simulink model "MPC_SinCasadi_V1_2016b"  (R2018b)
settings: Solver=ode4  StartTime=0.0  StopTime=inf  FixedStep=Ts  RelTol=1e-3
PreLoadFcn:
  | %% Parametros Simulacion %%
  | Ts = 50e-5; % tiempo simulacion
  | Tc = 2e-3;  % tiempo control
  | % Voltaje Nominal
  | vnom = 380;
  | % # de nodos
  | n = 4;
  | nic = 100;
  | pasoc = 0.1;
  | pv = 0.01;
  | px = 0.1;
  | 
  | % parametros de resistencia
  | r = [0.0226 0.0257 0.0769 0.0164 0.0513 0.0164 0.0411];
  | %Potencia Disponible
  | P = 100000;
  | %Bases de conversion
  | Vbase = 380;
  | Pbase = 1000;
  | %Filtros Droop
  | T = 0.5;
  | T1 = T;
  | T2 = T;
  | T3 = T;
  | T4 = T;
  | % Parametros del Droop
  | z1 = 0.0005527;
  | z2 = 0.0020;
  | z3 = 0.0017;
  | z4 = 0.0008107;
  | % Inicializacion Potencia y estados
  | Pi = 0.25;
  | xi = [Pi;Pi;Pi;Pi]*P;
  | % Filtro Potencia Disponible
  | Tf = 0.1;
  | % Filtro Control
  | Tfilter = 0.1;
InitFcn:
  | %% Parametros Simulacion %%
  | Ts = 50e-5; % tiempo simulacion
  | Tc = 2e-3;  % tiempo control
  | % Voltaje Nominal
  | vnom = 380;
  | % # de nodos
  | n = 4;
  | nic = 100;
  | pasoc = 0.1;
  | pv = 0.01;
  | px = 0.1;
  | 
  | % parametros de resistencia
  | r = [0.0226 0.0257 0.0769 0.0164 0.0513 0.0164 0.0411];
  | %Potencia Disponible
  | P = 100000;
  | %Bases de conversion
  | Vbase = 380;
  | Pbase = 1000;
  | %Filtros Droop
  | T = 0.5;
  | T1 = T;
  | T2 = T;
  | T3 = T;
  | T4 = T;
  | % Parametros del Droop
  | z1 = 0.0005527;
  | z2 = 0.0020;
  | z3 = 0.0017;
  | z4 = 0.0008107;
  | % Inicializacion Potencia y estados
  | Pi = 0.25;
  | xi = [Pi;Pi;Pi;Pi]*P;
  | % Filtro Potencia Disponible
  | Tf = 0.1;
  | % Filtro Control
  | Tfilter = 0.1;
undefined symbols (not defined in the file or in its folder): another_event_name, my_event_name
libraries: powerlib x38, rtlab x4, rtio_opalrt_common x3, simulink x1
settings Model: Creator=santi  LastModifiedBy=aperez
settings DataIOCC: ReturnWorkspaceOutputs=on
settings OptimizationCC: DefaultParameterBehavior=Inlined
settings DebuggingCC: UnconnectedInputMsg=none  UnconnectedOutputMsg=none  UnconnectedLineMsg=none  SFMachineParentedDataDiag=error
settings HardwareCC: TargetBitPerPointer=64  TargetBitPerSizeT=64  TargetBitPerPtrDiffT=64  TargetLongLongMode=on  TargetIntDivRoundTo=Zero  TargetEndianess=LittleEndian  TargetWordSize=64  TargetHWDeviceType=MATLAB Host  ProdEqTarget=off
settings ModelReferenceCC: EnableRefExpFcnMdlSchedulingChecks=off
settings RTWCC: SystemTargetFile=rtwsfcn.tlc  TemplateMakefile=rtwsfcn_default_tmf  Description=S-Function Target
settings CodeAppCC: StateflowObjectComments=on
settings STFCustomTargetCC: TargetLangStandard=C99 (ISO)  ModelReferenceCompliant=off  CompOptLevelCompliant=on  MATLABClassNameForMDSCustomization=Simulink.SoftwareTarget.TargetSpecificTriggerConfigurationBase  GRTInterface=on  SystemTargetFile=rtwsfcn.tlc

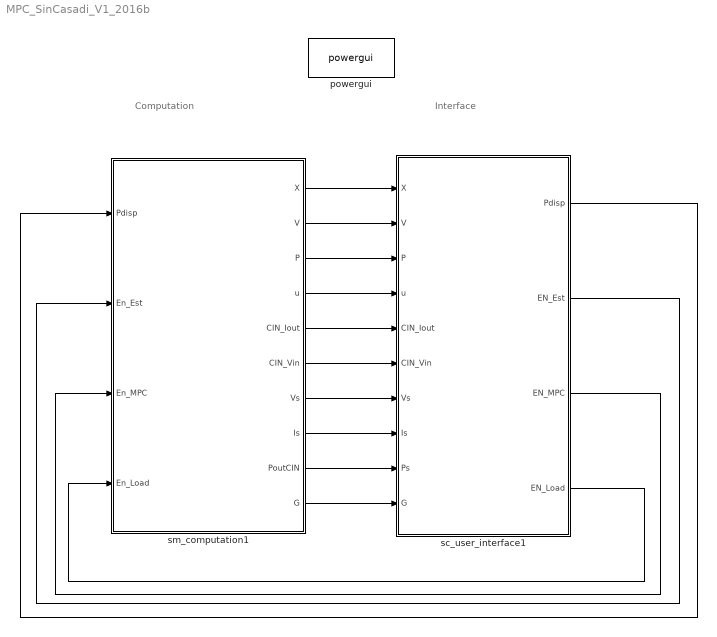
== system MPC_SinCasadi_V1_2016b ==
  note: Computation
  note: Interface
  powergui : powerlib/powergui  Priority=1  SimulationMode=Discrete  SampleTime=Ts  frequency=60  Iterations=50  frequencyindice=0  Pbase=100e6  ErrMax=1e-4  UnitsV=kV  UnitsW=MW  buscounter=0  FunctionMessages=off  echomessages=off  EnableUseOfTLC=off  CurrentSourceSwitches=off  DisableSnubberDevices=off  DisableRonSwitches=off  DisableVfSwitches=off  DisplayEquations=off  SolverType=Tustin/Backward Euler (TBE)  Interpol=off  ExternalGateDelay=off  methode=off  Ts=10  x0status=blocks  SPID=off  SwTol=0  HookPort=off  RestoreLinks=warning  ResistiveCurrentMeasurement=off  Frange=[0:2:500]  Ylog=off  Xlog=on  ShowGrid=off  save=off  variable=ZData  structure=0  ZoomFFT=off  StartTime=0.0  cycles=1  DisplayStyle=1  fundamental=60  FreqAxis=off  MaxFrequency=1000  frequencyindicesteady=1  RmsSteady=1  display=off
  sc_user_interface1 : Subsystem
  sm_computation1 : Subsystem
  wires:
  sc_user_interface1/1("Pdisp ") -> sm_computation1/1(Pdisp)
  sm_computation1/2(V) -> sc_user_interface1/2(V)
  sm_computation1/3(P) -> sc_user_interface1/3(P)
  sm_computation1/1(X) -> sc_user_interface1/1(X)
  sm_computation1/4(u) -> sc_user_interface1/4(u)
  sm_computation1/5(CIN_Iout) -> sc_user_interface1/5(CIN_Iout)
  sm_computation1/6(CIN_Vin) -> sc_user_interface1/6(CIN_Vin)
  sm_computation1/7(Vs) -> sc_user_interface1/7(Vs)
  sm_computation1/8(Is) -> sc_user_interface1/8(Is)
  sm_computation1/9(PoutCIN) -> sc_user_interface1/9(Ps)
  sm_computation1/10(G) -> sc_user_interface1/10(G)
  sc_user_interface1/2("EN_Est ") -> sm_computation1/2(En_Est)
  sc_user_interface1/3(EN_MPC) -> sm_computation1/3(En_MPC)
  sc_user_interface1/4("EN_Load ") -> sm_computation1/4(En_Load)

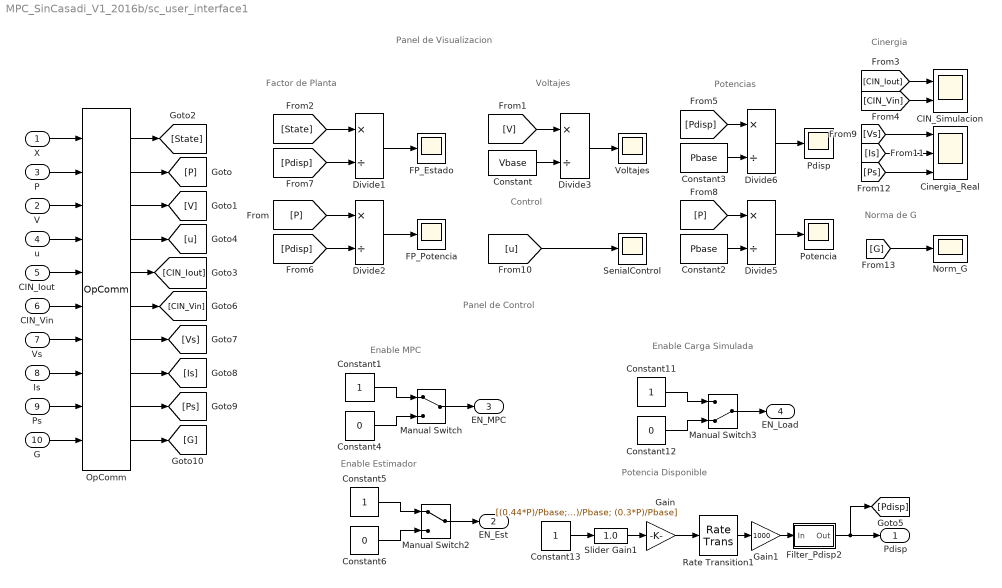
== system MPC_SinCasadi_V1_2016b/sc_user_interface1 ==
  note: Factor de Planta
  note: Potencias
  note: Voltajes
  note: Potencia Disponible
  note: Control
  note: Panel de Visualizacion
  note: Enable MPC
  note: Enable Estimador
  note: Enable Carga Simulada
  note: Panel de Control
  note: Cinergia
  note: Norma de G
  X : Inport
  V : Inport  Port=2
  P : Inport  Port=3
  u : Inport  Port=4
  CIN_Iout : Inport  Port=5
  CIN_Vin : Inport  Port=6
  Vs : Inport  Port=7
  Is : Inport  Port=8
  Ps : Inport  Port=9
  G : Inport  Port=10
  CIN_Simulacion : Scope  NumInputPorts=2
  Cinergia_Real : Scope  NumInputPorts=3
  Constant : Constant  Value=Vbase
  Constant{1,5,11,13} (4 alike) : Constant
  Constant12 : Constant  Value=0
  Constant2 : Constant  Value=Pbase
  Constant3 : Constant  Value=Pbase
  Constant4 : Constant  Value=0
  Constant6 : Constant  Value=0
  Divide{1..3,5..6} (5 alike) : Product  Inputs=*/
  FP_Estado : Scope
  FP_Potencia : Scope
  Filter_Pdisp2 : Subsystem
  Gain : Gain  Gain=[(0.44*P)/Pbase; (0.12*P)/Pbase; (0.14*P)/Pbase; (0.3*P)/Pbase]
  Gain1 : Gain  Gain=1000
  Manual Switch : ManualSwitch
  Manual Switch2 : ManualSwitch
  Manual Switch3 : ManualSwitch  CurrentSetting=0
  Norm_G : Scope
  OpComm : rtlab/OpComm  nbport=10  groupe_acq=1  subsys_rate=0  st=0  Synchronization=on  Interpolation=on  Threshold=1.0  Missed_Data=off  Sim_Time=off  Samples=off  dynSigOut=off  from_console=0  warning_done=off  writeOpCommFile=off  Offset=off
  Pdisp : Scope
  Potencia : Scope
  Rate Transition1 : RateTransition  InitialCondition=[45;12;20;30]  OutPortSampleTime=Tc
  SenialControl : Scope
  Slider Gain1 : simulink/Math Operations/Slider Gain  gain=1.0  low=0.4  high=1
  Voltajes : Scope
  "Pdisp " : Outport
  "EN_Est " : Outport  Port=2
  EN_MPC : Outport  Port=3
  "EN_Load " : Outport  Port=4
  wires:
  [P] -> Divide2/1
  Divide2/1 -> FP_Potencia/1
  Divide1/1 -> FP_Estado/1
  Divide3/1 -> Voltajes/1
  [V] -> Divide3/1
  Constant/1 -> Divide3/2
  [State] -> Divide1/1
  [Pdisp] -> Divide2/2
  [Pdisp] -> Divide1/2
  [P] -> Divide5/1
  Divide5/1 -> Potencia/1
  [u] -> SenialControl/1
  Constant2/1 -> Divide5/2
  Divide6/1 -> Pdisp/1
  Constant3/1 -> Divide6/2
  [Pdisp] -> Divide6/1
  X/1 -> OpComm/1
  P/1 -> OpComm/2
  V/1 -> OpComm/3
  OpComm/3 -> [V]
  OpComm/2 -> [P]
  OpComm/1 -> [State]
  OpComm/4 -> [u]
  u/1 -> OpComm/4
  Gain1/1 -> Filter_Pdisp2/1(In)
  Gain/1 -> Rate Transition1/1
  Filter_Pdisp2/1(Out) -> "Pdisp "/1, [Pdisp]
  Rate Transition1/1 -> Gain1/1
  CIN_Iout/1 -> OpComm/5
  CIN_Vin/1 -> OpComm/6
  Vs/1 -> OpComm/7
  Is/1 -> OpComm/8
  Ps/1 -> OpComm/9
  G/1 -> OpComm/10
  Constant1/1 -> Manual Switch/1
  Constant4/1 -> Manual Switch/2
  Manual Switch/1 -> EN_MPC/1
  Manual Switch2/1 -> "EN_Est "/1
  Constant6/1 -> Manual Switch2/2
  Constant5/1 -> Manual Switch2/1
  Constant11/1 -> Manual Switch3/1
  Constant12/1 -> Manual Switch3/2
  Manual Switch3/1 -> "EN_Load "/1
  Slider Gain1/1 -> Gain/1
  Constant13/1 -> Slider Gain1/1
  OpComm/5 -> [CIN_Iout]
  OpComm/6 -> [CIN_Vin]
  OpComm/7 -> [Vs]
  OpComm/8 -> [Is]
  OpComm/9 -> [Ps]
  OpComm/10 -> [G]
  [G] -> Norm_G/1
  [Vs] -> Cinergia_Real/1
  [Is] -> Cinergia_Real/2
  [Ps] -> Cinergia_Real/3
  [CIN_Vin] -> CIN_Simulacion/2
  [CIN_Iout] -> CIN_Simulacion/1

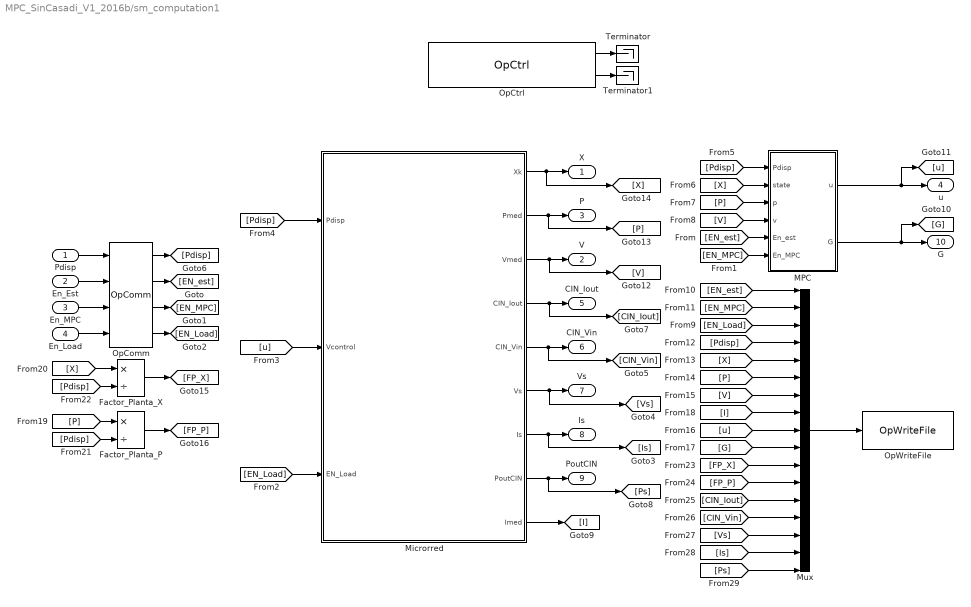
== system MPC_SinCasadi_V1_2016b/sm_computation1 ==
  Pdisp : Inport
  En_Est : Inport  Port=2
  En_MPC : Inport  Port=3
  En_Load : Inport  Port=4
  Factor_Planta_P : Product  Inputs=*/
  Factor_Planta_X : Product  Inputs=*/
  MPC : Subsystem
  Microrred : Subsystem
      settings: MinAlgLoopOccurrences=on
  Mux : Mux  Inputs=17
  OpComm : rtlab/OpComm  nbport=4  groupe_acq=1  subsys_rate=0  st=0  Synchronization=on  Interpolation=on  Threshold=1.0  Missed_Data=off  Sim_Time=off  Samples=off  dynSigOut=off  from_console=1  warning_done=off  writeOpCommFile=off  Offset=off
  OpCtrl : rtio_opalrt_common/OpCtrl  CtrlName='OpCtrl'  boardid=0  BitstreamFilename=VC707_2-EX-0001-3_2_3_354-eHSx128_C3C1FBCEC3C3FBFB-FF-01.bin  numconfig=-1  mode=Master  externalClock=off  decimRtsi=0  calibIO=off  SampleTime=Ts  loadinport=-1  BoardType=VC707  SecondaryPresent=off  sync_type=Audio
  OpWriteFile : rtlab/DataLogging/OpWriteFile  Static_File=on  varname=opvar  Filename=myfile.mat  rtpath='./'  nrtpath='.\'  Acq_Group=26  file_size=[]  write_offline=off  Sim_Mode=off  Nb_Samples=1000  Buffer_size=1000000
  Terminator : Terminator
  Terminator1 : Terminator
  X : Outport
  V : Outport  Port=2
  P : Outport  Port=3
  u : Outport  Port=4
  CIN_Iout : Outport  Port=5
  CIN_Vin : Outport  Port=6
  Vs : Outport  Port=7
  Is : Outport  Port=8
  PoutCIN : Outport  Port=9
  G : Outport  Port=10
  wires:
  Microrred/1(Xk) -> X/1, [X]
  Microrred/2(Pmed) -> [P], P/1
  Microrred/3(Vmed) -> V/1, [V]
  Pdisp/1 -> OpComm/1
  OpComm/1 -> [Pdisp]
  OpCtrl/1 -> Terminator/1
  OpCtrl/2 -> Terminator1/1
  MPC/1(u) -> [u], u/1
  Microrred/4(CIN_Iout) -> [CIN_Iout], CIN_Iout/1
  Microrred/6(Vs) -> Vs/1, [Vs]
  Microrred/8(PoutCIN) -> PoutCIN/1, [Ps]
  MPC/2(G) -> [G], G/1
  Microrred/7(Is) -> Is/1, [Is]
  Microrred/5(CIN_Vin) -> CIN_Vin/1, [CIN_Vin]
  En_Est/1 -> OpComm/2
  En_MPC/1 -> OpComm/3
  OpComm/2 -> [EN_est]
  OpComm/3 -> [EN_MPC]
  [EN_est] -> MPC/5(En_est)
  [EN_MPC] -> MPC/6(En_MPC)
  En_Load/1 -> OpComm/4
  OpComm/4 -> [EN_Load]
  [EN_Load] -> Microrred/3(EN_Load)
  Microrred/9(Imed) -> [I]
  [u] -> Microrred/2(Vcontrol)
  [Pdisp] -> Microrred/1(Pdisp)
  [Pdisp] -> MPC/1(Pdisp)
  [X] -> MPC/2(state)
  [P] -> MPC/3(p)
  [V] -> MPC/4(v)
  Mux/1 -> OpWriteFile/1
  [EN_est] -> Mux/1
  [EN_MPC] -> Mux/2
  [EN_Load] -> Mux/3
  [Pdisp] -> Mux/4
  [X] -> Mux/5
  [P] -> Mux/6
  [V] -> Mux/7
  [I] -> Mux/8
  [u] -> Mux/9
  [G] -> Mux/10
  [X] -> Factor_Planta_X/1
  [Pdisp] -> Factor_Planta_X/2
  [Pdisp] -> Factor_Planta_P/2
  [P] -> Factor_Planta_P/1
  Factor_Planta_X/1 -> [FP_X]
  Factor_Planta_P/1 -> [FP_P]
  [FP_X] -> Mux/11
  [FP_P] -> Mux/12
  [Ps] -> Mux/17
  [CIN_Iout] -> Mux/13
  [CIN_Vin] -> Mux/14
  [Vs] -> Mux/15
  [Is] -> Mux/16

== system MPC_SinCasadi_V1_2016b/sc_user_interface1/Filter_Pdisp2 ==
  In : Inport
  Demux : Demux
  Discrete Transfer Fcn{,1..3} (4 alike) : DiscreteTransferFcn  Denominator=[(Tf/Ts) -(Tf/Ts)+1]  InitialStates=0.25*P
  Mux7 : Mux
  Out : Outport
  wires:
  Demux/4 -> Discrete Transfer Fcn3/1
  Demux/3 -> Discrete Transfer Fcn2/1
  Discrete Transfer Fcn3/1 -> Mux7/4
  Demux/1 -> Discrete Transfer Fcn/1
  Discrete Transfer Fcn1/1 -> Mux7/2
  Demux/2 -> Discrete Transfer Fcn1/1
  Discrete Transfer Fcn/1 -> Mux7/1
  Discrete Transfer Fcn2/1 -> Mux7/3
  Mux7/1 -> Out/1
  In/1 -> Demux/1

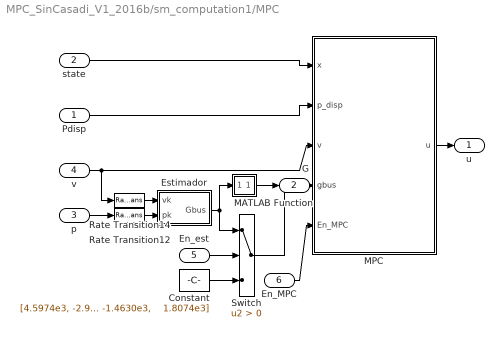
== system MPC_SinCasadi_V1_2016b/sm_computation1/MPC ==
  Pdisp : Inport
  state : Inport  Port=2
  p : Inport  Port=3
  v : Inport  Port=4
  En_est : Inport  Port=5
  En_MPC : Inport  Port=6
  Constant : Constant  Value="[4.5974e3, -2.9852e3, -1.2900e3, -0.3120e3; -2.9852e3, 2.9936e3, 0, 0; -1.2900e3,0,2.7560e3, -1.4630e3;   -0.3120e3,   0 ,  -1.4630e3,    1.8074e3]"
  Estimador : Subsystem
  MATLAB Function : MATLAB Function  TreatAsAtomicUnit=on
  MPC : Subsystem  TreatAsAtomicUnit=on  SystemSampleTime=Tc
      settings: MinAlgLoopOccurrences=on
  Rate Transition12 : RateTransition  InitialCondition=Pi*P  OutPortSampleTime=Tc
  Rate Transition14 : RateTransition  InitialCondition=[Vbase;Vbase;Vbase;Vbase]  OutPortSampleTime=Tc
  Switch : Switch  Criteria=u2 > Threshold
  u : Outport
  G : Outport  Port=2
  wires:
  Pdisp/1 -> MPC/2(p_disp)
  state/1 -> MPC/1(x)
  v/1 -> MPC/3(v), Rate Transition14/1
  p/1 -> Rate Transition12/1
  Rate Transition14/1 -> Estimador/1(vk)
  Rate Transition12/1 -> Estimador/2(pk)
  MPC/1(u) -> u/1
  En_est/1 -> Switch/2
  Switch/1 -> MPC/4(gbus)
  Estimador/1(Gbus) -> Switch/1, MATLAB Function/1(G)
  Constant/1 -> Switch/3
  MATLAB Function/1(normG) -> G/1
  En_MPC/1 -> MPC/5(En_MPC)

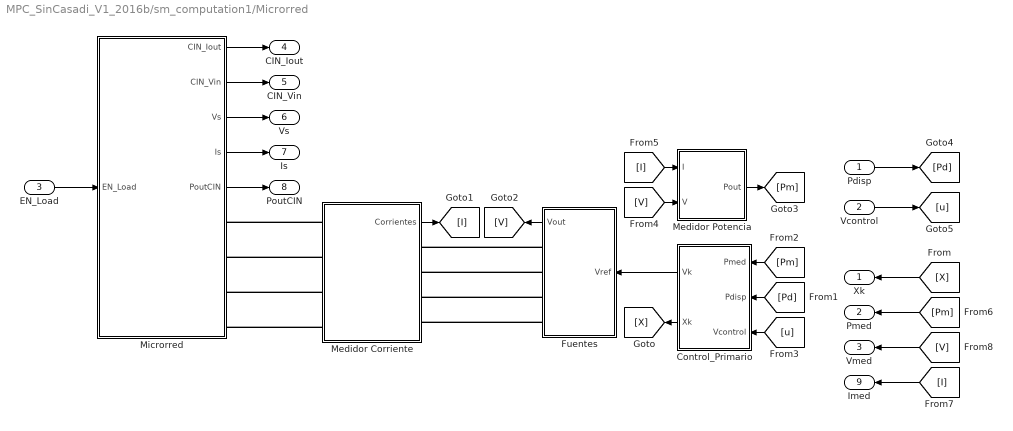
== system MPC_SinCasadi_V1_2016b/sm_computation1/Microrred ==
  Pdisp : Inport
  Vcontrol : Inport  Port=2
  EN_Load : Inport  Port=3
  Control_Primario : Subsystem
  Fuentes : Subsystem
  Medidor Corriente : Subsystem
  Medidor Potencia : Subsystem
  Microrred : Subsystem
  Xk : Outport
  Pmed : Outport  Port=2
  Vmed : Outport  Port=3
  CIN_Iout : Outport  Port=4
  CIN_Vin : Outport  Port=5
  Vs : Outport  Port=6
  Is : Outport  Port=7
  PoutCIN : Outport  Port=8
  Imed : Outport  Port=9
  wires:
  Control_Primario/1(Vk) -> Fuentes/1(Vref)
  Control_Primario/2(Xk) -> [X]
  Medidor Corriente/1(Corrientes) -> [I]
  Fuentes/1(Vout) -> [V]
  [Pd] -> Control_Primario/2(Pdisp)
  [Pm] -> Control_Primario/1(Pmed)
  [u] -> Control_Primario/3(Vcontrol)
  [V] -> Medidor Potencia/2(V)
  [I] -> Medidor Potencia/1(I)
  Medidor Potencia/1(Pout) -> [Pm]
  [X] -> Xk/1
  [Pm] -> Pmed/1
  [V] -> Vmed/1
  Pdisp/1 -> [Pd]
  Vcontrol/1 -> [u]
  Microrred/1(CIN_Iout) -> CIN_Iout/1
  Microrred/2(CIN_Vin) -> CIN_Vin/1
  Microrred/3(Vs) -> Vs/1
  Microrred/4(Is) -> Is/1
  Microrred/5(PoutCIN) -> PoutCIN/1
  EN_Load/1 -> Microrred/1(EN_Load)
  [I] -> Imed/1
  connections:
  Fuentes/RConn3 -- Medidor Corriente/RConn3
  Medidor Corriente/LConn3 -- Microrred/RConn3
  Fuentes/RConn4 -- Medidor Corriente/RConn4
  Medidor Corriente/LConn2 -- Microrred/RConn2
  Fuentes/RConn1 -- Medidor Corriente/RConn1
  Medidor Corriente/LConn1 -- Microrred/RConn1
  Fuentes/RConn2 -- Medidor Corriente/RConn2
  Medidor Corriente/LConn4 -- Microrred/RConn4

== system MPC_SinCasadi_V1_2016b/sm_computation1/MPC/Estimador ==
  vk : Inport
  pk : Inport  Port=2
  MATLAB System : MATLABSystem  System=Estimador_pu  Vbase=Vbase  Pbase=Pbase  SimulateUsing=Code generation
      mask Type: Estimador_pu
      mask Display:
      | disp('Estimador_pu');
      | port_label('input',1,'vk');
      | port_label('input',2,'pk');
      | port_label('output',1,'Gbus');
  Gbus : Outport
  wires:
  pk/1 -> MATLAB System/2
  vk/1 -> MATLAB System/1
  MATLAB System/1 -> Gbus/1

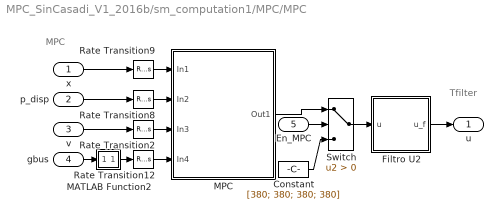
== system MPC_SinCasadi_V1_2016b/sm_computation1/MPC/MPC ==
  note: MPC
  note: Tfilter
  x : Inport
  p_disp : Inport  Port=2
  v : Inport  Port=3
  gbus : Inport  Port=4
  En_MPC : Inport  Port=5
  Constant : Constant  Value=[380; 380; 380; 380]
  Filtro U2 : Subsystem
  MATLAB Function2 : MATLAB Function  TreatAsAtomicUnit=on
  MPC : Subsystem  SystemSampleTime=2e-3
  Rate Transition12 : RateTransition  InitialCondition="[4.5974e3, -2.9852e3, -1.2900e3, -0.3120e3, -2.9852e3, 2.9936e3, 0, 0, -1.2900e3,0,2.7560e3, -1.4630e3,   -0.3120e3,   0 ,  -1.4630e3,    1.8074e3]"  OutPortSampleTime=Tc
  Rate Transition2 : RateTransition  InitialCondition=[Vbase;Vbase;Vbase;Vbase]  OutPortSampleTime=Tc
  Rate Transition8 : RateTransition  InitialCondition=Pi*P  OutPortSampleTime=Tc
  Rate Transition9 : RateTransition  InitialCondition=Pi*P  OutPortSampleTime=Tc
  Switch : Switch  Criteria=u2 > Threshold
  u : Outport
  wires:
  p_disp/1 -> Rate Transition8/1
  x/1 -> Rate Transition9/1
  v/1 -> Rate Transition2/1
  gbus/1 -> MATLAB Function2/1(gbus)
  Filtro U2/1(u_f) -> u/1
  Rate Transition9/1 -> MPC/1(In1)
  Rate Transition8/1 -> MPC/2(In2)
  Rate Transition2/1 -> MPC/3(In3)
  Rate Transition12/1 -> MPC/4(In4)
  MATLAB Function2/1(G) -> Rate Transition12/1
  MPC/1(Out1) -> Switch/1
  Switch/1 -> Filtro U2/1(u)
  Constant/1 -> Switch/3
  En_MPC/1 -> Switch/2

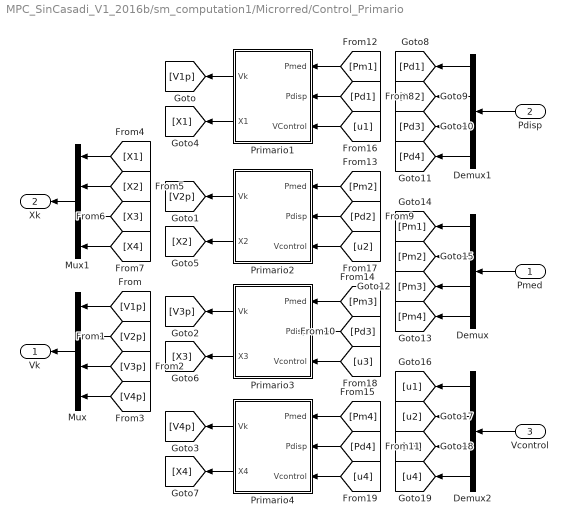
== system MPC_SinCasadi_V1_2016b/sm_computation1/Microrred/Control_Primario ==
  Pmed : Inport
  Pdisp : Inport  Port=2
  Vcontrol : Inport  Port=3
  Demux : Demux
  Demux1 : Demux
  Demux2 : Demux
  Mux : Mux
  Mux1 : Mux
  Primario1 : Subsystem
  Primario2 : Subsystem
  Primario3 : Subsystem
  Primario4 : Subsystem
  Vk : Outport
  Xk : Outport  Port=2
  wires:
  Vcontrol/1 -> Demux2/1
  Mux1/1 -> Xk/1
  Pmed/1 -> Demux/1
  Mux/1 -> Vk/1
  Pdisp/1 -> Demux1/1
  Primario1/1(Vk) -> [V1p]
  [V1p] -> Mux/1
  [V2p] -> Mux/2
  [V3p] -> Mux/3
  [V4p] -> Mux/4
  Primario2/1(Vk) -> [V2p]
  Primario3/1(Vk) -> [V3p]
  Primario4/1(Vk) -> [V4p]
  [X1] -> Mux1/1
  [X2] -> Mux1/2
  [X3] -> Mux1/3
  [X4] -> Mux1/4
  Primario2/2(X2) -> [X2]
  Primario3/2(X3) -> [X3]
  Primario4/2(X4) -> [X4]
  Primario1/2(X1) -> [X1]
  Demux1/1 -> [Pd1]
  Demux1/2 -> [Pd2]
  Demux1/3 -> [Pd3]
  Demux1/4 -> [Pd4]
  [Pd1] -> Primario1/2(Pdisp)
  [Pd2] -> Primario2/2(Pdisp)
  [Pd3] -> Primario3/2(Pdisp)
  [Pd4] -> Primario4/2(Pdisp)
  Demux/1 -> [Pm1]
  Demux/2 -> [Pm2]
  Demux/3 -> [Pm3]
  Demux/4 -> [Pm4]
  [Pm1] -> Primario1/1(Pmed)
  [Pm2] -> Primario2/1(Pmed)
  [Pm3] -> Primario3/1(Pmed)
  [Pm4] -> Primario4/1(Pmed)
  Demux2/1 -> [u1]
  Demux2/2 -> [u2]
  Demux2/3 -> [u3]
  Demux2/4 -> [u4]
  [u4] -> Primario4/3(Vcontrol)
  [u3] -> Primario3/3(Vcontrol)
  [u2] -> Primario2/3(Vcontrol)
  [u1] -> Primario1/3(VControl)

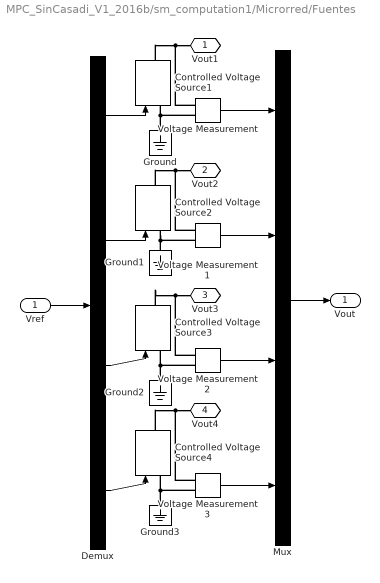
== system MPC_SinCasadi_V1_2016b/sm_computation1/Microrred/Fuentes ==
  Vref : Inport
  Controlled Voltage Source{1..4} (4 alike) : powerlib/Electrical Sources/Controlled Voltage Source  Initialize=on  Source_Type=DC  Amplitude=vnom  Phase=0  Frequency=0  Measurements=None
  Demux : Demux
  Ground{,1..3} (4 alike) : powerlib/Elements/Ground  LConnTagsString=a
  Mux : Mux
  Voltage Measurement{,1..3} (4 alike) : powerlib/Measurements/Voltage Measurement  PhasorSimulation=off  OutputType=Complex  PSBequivalent=0
  Vout1 : PMIOPort  Side=Right
  Vout2 : PMIOPort  Port=2  Side=Right
  Vout3 : PMIOPort  Port=3  Side=Right
  Vout4 : PMIOPort  Port=4  Side=Right
  Vout : Outport
  wires:
  Mux/1 -> Vout/1
  Voltage Measurement2/1 -> Mux/3
  Voltage Measurement1/1 -> Mux/2
  Voltage Measurement3/1 -> Mux/4
  Voltage Measurement/1 -> Mux/1
  Vref/1 -> Demux/1
  Demux/4 -> Controlled Voltage Source4/1
  Demux/3 -> Controlled Voltage Source3/1
  Demux/2 -> Controlled Voltage Source2/1
  Demux/1 -> Controlled Voltage Source1/1
  connections:
  Vout4/RConn1 -- Voltage Measurement3/LConn1 -- Controlled Voltage Source4/RConn1
  Voltage Measurement3/LConn2 -- Ground3/LConn1 -- Controlled Voltage Source4/LConn1
  Voltage Measurement2/LConn2 -- Ground2/LConn1 -- Controlled Voltage Source3/LConn1
  Vout3/RConn1 -- Voltage Measurement2/LConn1 -- Controlled Voltage Source3/RConn1
  Vout2/RConn1 -- Voltage Measurement1/LConn1 -- Controlled Voltage Source2/RConn1
  Voltage Measurement1/LConn2 -- Controlled Voltage Source2/LConn1 -- Ground1/LConn1
  Voltage Measurement/LConn2 -- Controlled Voltage Source1/LConn1 -- Ground/LConn1
  Vout1/RConn1 -- Voltage Measurement/LConn1 -- Controlled Voltage Source1/RConn1

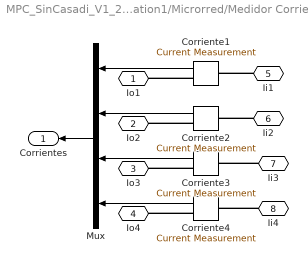
== system MPC_SinCasadi_V1_2016b/sm_computation1/Microrred/Medidor Corriente ==
  Corriente{1..4} (4 alike) : powerlib/Measurements/Current Measurement  PhasorSimulation=off  OutputType=Complex  PSBequivalent=0
  Mux : Mux
  Io1 : PMIOPort  Side=Left
  Io2 : PMIOPort  Port=2  Side=Left
  Io3 : PMIOPort  Port=3  Side=Left
  Io4 : PMIOPort  Port=4  Side=Left
  Ii1 : PMIOPort  Port=5  Side=Right
  Ii2 : PMIOPort  Port=6  Side=Right
  Ii3 : PMIOPort  Port=7  Side=Right
  Ii4 : PMIOPort  Port=8  Side=Right
  Corrientes : Outport
  wires:
  Mux/1 -> Corrientes/1
  Corriente3/1 -> Mux/3
  Corriente2/1 -> Mux/2
  Corriente4/1 -> Mux/4
  Corriente1/1 -> Mux/1
  connections:
  Corriente4/RConn1 -- Io4/RConn1
  Corriente3/RConn1 -- Io3/RConn1
  Corriente2/RConn1 -- Io2/RConn1
  Corriente1/RConn1 -- Io1/RConn1
  Ii4/RConn1 -- Corriente4/LConn1
  Ii3/RConn1 -- Corriente3/LConn1
  Ii2/RConn1 -- Corriente2/LConn1
  Ii1/RConn1 -- Corriente1/LConn1

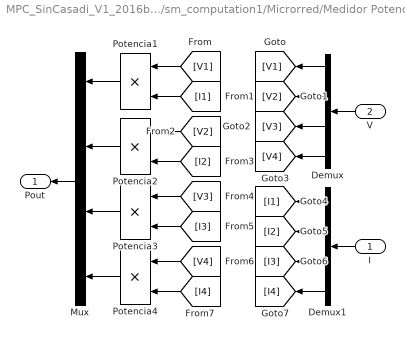
== system MPC_SinCasadi_V1_2016b/sm_computation1/Microrred/Medidor Potencia ==
  I : Inport
  V : Inport  Port=2
  Demux : Demux
  Demux1 : Demux
  Mux : Mux
  Potencia{1..4} (4 alike) : Product
  Pout : Outport
  wires:
  I/1 -> Demux1/1
  V/1 -> Demux/1
  Potencia3/1 -> Mux/3
  Potencia2/1 -> Mux/2
  Potencia1/1 -> Mux/1
  Potencia4/1 -> Mux/4
  Mux/1 -> Pout/1
  Demux/1 -> [V1]
  Demux/2 -> [V2]
  Demux/3 -> [V3]
  Demux/4 -> [V4]
  Demux1/1 -> [I1]
  Demux1/2 -> [I2]
  Demux1/3 -> [I3]
  Demux1/4 -> [I4]
  [V1] -> Potencia1/1
  [I1] -> Potencia1/2
  [V2] -> Potencia2/1
  [I2] -> Potencia2/2
  [V3] -> Potencia3/1
  [I3] -> Potencia3/2
  [V4] -> Potencia4/1
  [I4] -> Potencia4/2

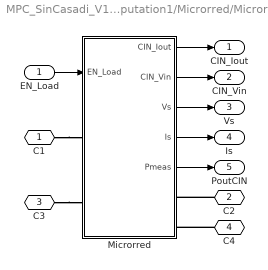
== system MPC_SinCasadi_V1_2016b/sm_computation1/Microrred/Microrred ==
  EN_Load : Inport
  Microrred : Subsystem
  C1 : PMIOPort  Side=Right
  C2 : PMIOPort  Port=2  Side=Right
  C3 : PMIOPort  Port=3  Side=Right
  C4 : PMIOPort  Port=4  Side=Right
  CIN_Iout : Outport
  CIN_Vin : Outport  Port=2
  Vs : Outport  Port=3
  Is : Outport  Port=4
  PoutCIN : Outport  Port=5
  wires:
  Microrred/1(CIN_Iout) -> CIN_Iout/1
  Microrred/2(CIN_Vin) -> CIN_Vin/1
  Microrred/3(Vs) -> Vs/1
  Microrred/4(Is) -> Is/1
  Microrred/5(Pmeas) -> PoutCIN/1
  EN_Load/1 -> Microrred/1(EN_Load)
  connections:
  C1/RConn1 -- Microrred/LConn1
  C3/RConn1 -- Microrred/LConn2
  C2/RConn1 -- Microrred/RConn1
  C4/RConn1 -- Microrred/RConn2

== system MPC_SinCasadi_V1_2016b/sm_computation1/MPC/MPC/Filtro U2 ==
  u : Inport
  Demux : Demux
  Discrete Transfer Fcn{,1..3} (4 alike) : DiscreteTransferFcn  Denominator=[(Tfilter/Ts) -(Tfilter/Ts)+1]  InitialStates=vnom
  Mux : Mux
  u_f : Outport
  wires:
  Discrete Transfer Fcn/1 -> Mux/1
  Discrete Transfer Fcn3/1 -> Mux/4
  Discrete Transfer Fcn1/1 -> Mux/2
  Discrete Transfer Fcn2/1 -> Mux/3
  Demux/1 -> Discrete Transfer Fcn/1
  Demux/4 -> Discrete Transfer Fcn3/1
  Demux/2 -> Discrete Transfer Fcn1/1
  Demux/3 -> Discrete Transfer Fcn2/1
  u/1 -> Demux/1
  Mux/1 -> u_f/1

== system MPC_SinCasadi_V1_2016b/sm_computation1/MPC/MPC/MPC ==
  In1 : Inport
  In2 : Inport  Port=2
  In3 : Inport  Port=3
  In4 : Inport  Port=4
  MPC : S-Function  FunctionName=MPC_Params  Parameters=Tc,n,nic,pasoc,pv,Vbase,Pbase,T1,T2,T3,T4,z1,z2,z3,z4,px  SFunctionModules='MPC_Params_wrapper'  SFunctionDeploymentMode=off  EnableBusSupport=off
  Out1 : Outport
  wires:
  In4/1 -> MPC/4
  In1/1 -> MPC/1
  MPC/1 -> Out1/1
  In3/1 -> MPC/3
  In2/1 -> MPC/2

== system MPC_SinCasadi_V1_2016b/sm_computation1/Microrred/Control_Primario/Primario1 ==
  note: Vcontrol
  note: Pdisponible
  Pmed : Inport
  Pdisp : Inport  Port=2
  VControl : Inport  Port=3
  Discrete Transfer Fcn : DiscreteTransferFcn  Denominator=[(T1/Ts) -(T1/Ts)+1]  InitialStates=xi(1)
  Gain : Gain  Gain=z1
  Sum : Sum  Inputs=|-+
  Sum1 : Sum  Inputs=|++
  Vk : Outport
  X1 : Outport  Port=2
  wires:
  Discrete Transfer Fcn/1 -> X1/1, Sum/1
  Sum/1 -> Gain/1
  Gain/1 -> Sum1/1
  VControl/1 -> Sum1/2
  Pmed/1 -> Discrete Transfer Fcn/1
  Pdisp/1 -> Sum/2
  Sum1/1 -> Vk/1

== system MPC_SinCasadi_V1_2016b/sm_computation1/Microrred/Control_Primario/Primario2 ==
  note: Pdisponible
  note: Vcontrol
  Pmed : Inport
  Pdisp : Inport  Port=2
  Vcontrol : Inport  Port=3
  Discrete Transfer Fcn : DiscreteTransferFcn  Denominator=[(T2/Ts) -(T1/Ts)+1]  InitialStates=xi(2)
  Display : Display
  Gain : Gain  Gain=z2
  Sum : Sum  Inputs=|-+
  Sum1 : Sum  Inputs=|++
  Vk : Outport
  X2 : Outport  Port=2
  wires:
  Sum1/1 -> Vk/1
  Pdisp/1 -> Sum/2
  Pmed/1 -> Discrete Transfer Fcn/1
  Vcontrol/1 -> Sum1/2
  Gain/1 -> Display/1, Sum1/1
  Sum/1 -> Gain/1
  Discrete Transfer Fcn/1 -> X2/1, Sum/1

== system MPC_SinCasadi_V1_2016b/sm_computation1/Microrred/Control_Primario/Primario3 ==
  note: Vcontrol
  note: Pdisponible
  Pmed : Inport
  Pdisp : Inport  Port=2
  Vcontrol : Inport  Port=3
  Discrete Transfer Fcn : DiscreteTransferFcn  Denominator=[(T3/Ts) -(T1/Ts)+1]  InitialStates=xi(3)
  Gain : Gain  Gain=z3
  Sum : Sum  Inputs=|-+
  Sum1 : Sum  Inputs=|++
  Vk : Outport
  X3 : Outport  Port=2
  wires:
  Sum/1 -> Gain/1
  Gain/1 -> Sum1/1
  Vcontrol/1 -> Sum1/2
  Pmed/1 -> Discrete Transfer Fcn/1
  Pdisp/1 -> Sum/2
  Discrete Transfer Fcn/1 -> Sum/1, X3/1
  Sum1/1 -> Vk/1

== system MPC_SinCasadi_V1_2016b/sm_computation1/Microrred/Control_Primario/Primario4 ==
  note: Pdisponible
  note: Vcontrol
  Pmed : Inport
  Pdisp : Inport  Port=2
  Vcontrol : Inport  Port=3
  Discrete Transfer Fcn : DiscreteTransferFcn  Denominator=[(T4/Ts) -(T1/Ts)+1]  InitialStates=xi(4)
  Gain : Gain  Gain=z4
  Sum : Sum  Inputs=|-+
  Sum1 : Sum  Inputs=|++
  Vk : Outport
  X4 : Outport  Port=2
  wires:
  Sum1/1 -> Vk/1
  Discrete Transfer Fcn/1 -> Sum/1, X4/1
  Pdisp/1 -> Sum/2
  Pmed/1 -> Discrete Transfer Fcn/1
  Vcontrol/1 -> Sum1/2
  Gain/1 -> Sum1/1
  Sum/1 -> Gain/1

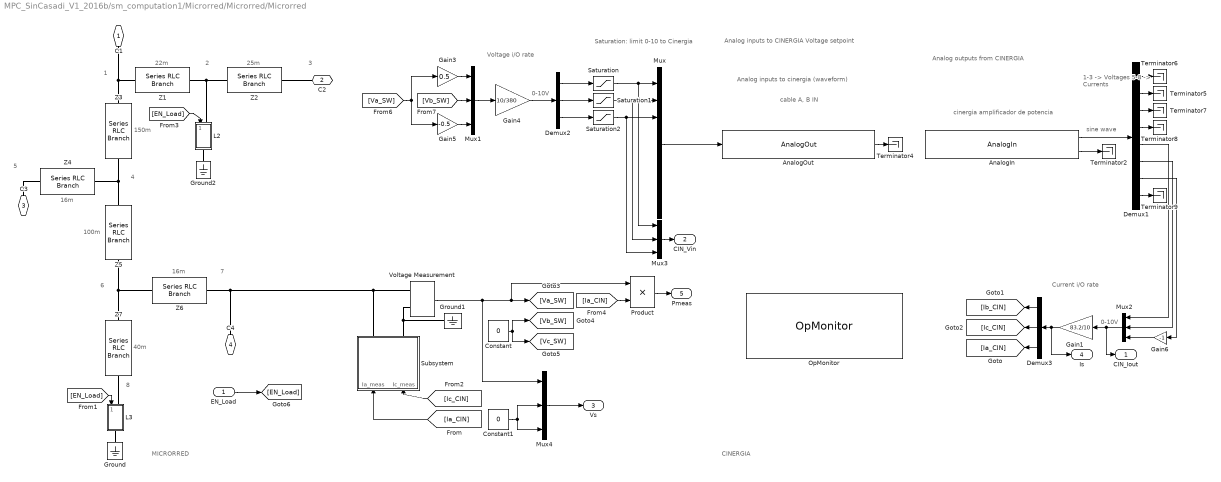
== system MPC_SinCasadi_V1_2016b/sm_computation1/Microrred/Microrred/Microrred ==
  note: MICRORRED
  note: 22m
  note: 8
  note: 7
  note: 6
  note: 5
  note: 4
  note: 1
  note: 2
  note: 3
  note: 25m
  note: 150m
  note: 16m
  note: 100m
  note: 16m
  note: 40m
  note: cable A, B IN
  note: 0-10V
  note: 1-3 -> Voltages
      | 5-8 -> Currents
  note: Analog inputs to cinergia (waveform)
  note: Current i/O rate
  note: sine wave
  note: Analog outputs from CINERGIA
  note: Voltage i/O rate
  note: cinergia amplificador de potencia
  note: 0-10V
  note: Saturation: limit 0-10 to Cinergia
  note: Analog inputs to CINERGIA
      | Voltage setpoint
  note: CINERGIA
  EN_Load : Inport
  AnalogIn : rtio_opalrt_common/AnalogIn  CtrlName='OpCtrl'  portNb=11  FcnNos=Slot 1 Module B Subsection 1  size=16  maxcount=8  count=8  numchan=8  sampleTime=Ts
      settings: AttributesFormatString=%<CtrlName>
  AnalogOut : rtio_opalrt_common/AnalogOut  CtrlName='OpCtrl'  portNb=19  FcnNos=Slot 1 Module A Subsection 1  size=32  maxcount=8  count=8  numchan=8  israngeinput=off  voltagerange=[-10 ... 10]  slot=0  side=0  mismatch=0  slotside=Slot_1_Module_A
      settings: AttributesFormatString=%<CtrlName>
  Constant : Constant  Value=0
  Constant1 : Constant  Value=0
  Demux1 : Demux  Outputs=8
  Demux2 : Demux  Outputs=3
  Demux3 : Demux  Outputs=3
  Gain1 : Gain  Gain=83.2/10
  Gain3 : Gain  Gain=0.5
  Gain4 : Gain  Gain=10/380
  Gain5 : Gain  Gain=-0.5
  Gain6 : Gain  Gain=-1
  Ground : powerlib/Elements/Ground  LConnTagsString=a
  Ground1 : powerlib/Elements/Ground  LConnTagsString=a
  Ground2 : powerlib/Elements/Ground  LConnTagsString=a
  L2 : Subsystem
      settings: MinAlgLoopOccurrences=on
  L3 : Subsystem
      settings: MinAlgLoopOccurrences=on
  Mux : Mux  Inputs=8
  Mux{1..4} (4 alike) : Mux  Inputs=3
  OpMonitor : rtlab/Monitoring/OpMonitor  compute_time=on  real_step=on  idle_time=on  nb_overruns=on  user_time=off  user_name=my_event_name,another_event_name
  Product : Product
  Saturation : Saturate  UpperLimit=10  LowerLimit=-10
  Saturation1 : Saturate  UpperLimit=10  LowerLimit=-10
  Saturation2 : Saturate  UpperLimit=10  LowerLimit=-10
  Subsystem : Subsystem
  Terminator{2,4..9} (7 alike) : Terminator
  Voltage Measurement : powerlib/Measurements/Voltage Measurement  PhasorSimulation=off  OutputType=Complex  PSBequivalent=0
  Z1 : powerlib/Elements/Series RLC Branch  LConnTagsString=__new0  RConnTagsString=__new0  BranchType=RL  Resistance=r(1)  Inductance=433e-6  SetiL0=off  InitialCurrent=0  Capacitance=1e-6  Setx0=off  InitialVoltage=0  Measurements=None
  Z2 : powerlib/Elements/Series RLC Branch  LConnTagsString=__new0  RConnTagsString=__new0  BranchType=RL  Resistance=r(2)  Inductance=500e-6  SetiL0=off  InitialCurrent=0  Capacitance=1e-6  Setx0=off  InitialVoltage=0  Measurements=None
  Z3 : powerlib/Elements/Series RLC Branch  LConnTagsString=__new0  RConnTagsString=__new0  BranchType=RL  Resistance=r(3)  Inductance=34e-6  SetiL0=off  InitialCurrent=0  Capacitance=1e-6  Setx0=off  InitialVoltage=0  Measurements=None
  Z4 : powerlib/Elements/Series RLC Branch  LConnTagsString=__new0  RConnTagsString=__new0  BranchType=RL  Resistance=r(4)  Inductance=609e-6  SetiL0=off  InitialCurrent=0  Capacitance=1e-6  Setx0=off  InitialVoltage=0  Measurements=None
  Z5 : powerlib/Elements/Series RLC Branch  LConnTagsString=__new0  RConnTagsString=__new0  BranchType=RL  Resistance=r(5)  Inductance=22e-6  SetiL0=off  InitialCurrent=0  Capacitance=1e-6  Setx0=off  InitialVoltage=0  Measurements=None
  Z6 : powerlib/Elements/Series RLC Branch  LConnTagsString=__new0  RConnTagsString=__new0  BranchType=RL  Resistance=r(6)  Inductance=305e-6  SetiL0=off  InitialCurrent=0  Capacitance=1e-6  Setx0=off  InitialVoltage=0  Measurements=None
  Z7 : powerlib/Elements/Series RLC Branch  LConnTagsString=__new0  RConnTagsString=__new0  BranchType=RL  Resistance=r(7)  Inductance=836e-6  SetiL0=off  InitialCurrent=0  Capacitance=1e-6  Setx0=off  InitialVoltage=0  Measurements=None
  C1 : PMIOPort  Side=Left
  C2 : PMIOPort  Port=2  Side=Right
  C3 : PMIOPort  Port=3  Side=Left
  C4 : PMIOPort  Port=4  Side=Right
  CIN_Iout : Outport
  CIN_Vin : Outport  Port=2
  Vs : Outport  Port=3
  Is : Outport  Port=4
  Pmeas : Outport  Port=5
  wires:
  Demux1/3 -> Terminator7/1
  Demux1/8 -> Terminator9/1
  Demux2/1 -> Saturation/1
  [Ic_CIN] -> Subsystem/2(Ic_meas)
  [Va_SW] -> Gain3/1, Gain5/1
  Mux/1 -> AnalogOut/1
  [Vb_SW] -> Mux1/2
  Demux2/3 -> Saturation2/1
  Mux3/1 -> CIN_Vin/1
  Gain4/1 -> Demux2/1
  Constant/1 -> [Vb_SW], [Vc_SW]
  AnalogOut/1 -> Terminator4/1
  Saturation2/1 -> Mux3/3, Mux/3
  Demux1/4 -> Terminator8/1
  Demux2/2 -> Saturation1/1
  Saturation/1 -> Mux3/1, Mux/1
  Saturation1/1 -> Mux3/2, Mux/2
  Demux1/1 -> Terminator6/1
  Demux1/6 -> Mux2/2
  Demux1/7 -> Gain6/1
  Mux2/1 -> CIN_Iout/1, Gain1/1
  [Ia_CIN] -> Subsystem/1(Ia_meas)
  Demux1/2 -> Terminator5/1
  Gain1/1 -> Is/1, Demux3/1
  AnalogIn/2 -> Terminator2/1
  AnalogIn/1 -> Demux1/1
  Mux4/1 -> Vs/1
  Voltage Measurement/1 -> Product/1, [Va_SW], Mux4/1
  Product/1 -> Pmeas/1
  Mux1/1 -> Gain4/1
  Gain3/1 -> Mux1/1
  Gain5/1 -> Mux1/3
  Demux1/5 -> Mux2/1
  Gain6/1 -> Mux2/3
  Demux3/1 -> [Ib_CIN]
  Demux3/3 -> [Ia_CIN]
  Demux3/2 -> [Ic_CIN]
  EN_Load/1 -> [EN_Load]
  [EN_Load] -> L3/1("L3 ")
  [EN_Load] -> L2/1(L2)
  [Ia_CIN] -> Product/2
  Constant1/1 -> Mux4/2, Mux4/3
  connections:
  Z4/LConn1 -- Z5/RConn1 -- Z3/RConn1
  C3/RConn1 -- Z4/RConn1
  Z5/LConn1 -- Z7/LConn1 -- Z6/LConn1
  Z1/RConn1 -- L2/LConn1 -- Z2/LConn1
  C2/RConn1 -- Z2/RConn1
  Z3/LConn1 -- C1/RConn1 -- Z1/LConn1
  L3/LConn1 -- Z7/RConn1
  Ground/LConn1 -- L3/RConn1
  Ground2/LConn1 -- L2/RConn1
  Z6/RConn1 -- C4/RConn1 -- Subsystem/RConn1 -- Voltage Measurement/LConn1
  Subsystem/RConn2 -- Voltage Measurement/LConn2 -- Ground1/LConn1

== system MPC_SinCasadi_V1_2016b/sm_computation1/Microrred/Microrred/Microrred/L2 ==
  L2 : Inport
  Constant : Constant
  Constant1 : Constant  Value=0
  Ideal Switch : powerlib/Power Electronics/Ideal Switch  Ron=0.001  Lon=0  IC=0  Rs=1e5  Cs=inf  Measurements=off
  Series RLC Branch : powerlib/Elements/Series RLC Branch  LConnTagsString=__new0  RConnTagsString=__new0  BranchType=R  Resistance=14.44  Inductance=1e-3  SetiL0=off  InitialCurrent=0  Capacitance=1e-6  Setx0=off  InitialVoltage=0  Measurements=None
  Series RLC Branch3 : powerlib/Elements/Series RLC Branch  LConnTagsString=__new0  RConnTagsString=__new0  BranchType=R  Resistance=72.2  Inductance=1e-3  SetiL0=off  InitialCurrent=0  Capacitance=1e-6  Setx0=off  InitialVoltage=0  Measurements=None
  Switch : Switch  Criteria=u2 > Threshold
  + : PMIOPort  Side=Left
  - : PMIOPort  Port=2  Side=Right
  wires:
  Constant1/1 -> Switch/3
  Switch/1 -> Ideal Switch/1
  Constant/1 -> Switch/1
  L2/1 -> Switch/2
  connections:
  Series RLC Branch3/LConn1 -- Ideal Switch/LConn1
  Series RLC Branch/RConn1 -- Series RLC Branch3/RConn1 -- -/RConn1
  Ideal Switch/RConn1 -- +/RConn1 -- Series RLC Branch/LConn1

== system MPC_SinCasadi_V1_2016b/sm_computation1/Microrred/Microrred/Microrred/L3 ==
  "L3 " : Inport
  Constant : Constant
  Constant1 : Constant  Value=0
  Ideal Switch : powerlib/Power Electronics/Ideal Switch  Ron=0.001  Lon=0  IC=0  Rs=1e5  Cs=inf  Measurements=off
  Series RLC Branch : powerlib/Elements/Series RLC Branch  LConnTagsString=__new0  RConnTagsString=__new0  BranchType=R  Resistance=18.05  Inductance=1e-3  SetiL0=off  InitialCurrent=0  Capacitance=1e-6  Setx0=off  InitialVoltage=0  Measurements=None
  Series RLC Branch3 : powerlib/Elements/Series RLC Branch  LConnTagsString=__new0  RConnTagsString=__new0  BranchType=R  Resistance=96.26  Inductance=1e-3  SetiL0=off  InitialCurrent=0  Capacitance=1e-6  Setx0=off  InitialVoltage=0  Measurements=None
  Switch : Switch  Criteria=u2 > Threshold
  + : PMIOPort  Side=Left
  - : PMIOPort  Port=2  Side=Right
  wires:
  Constant1/1 -> Switch/3
  Switch/1 -> Ideal Switch/1
  Constant/1 -> Switch/1
  "L3 "/1 -> Switch/2
  connections:
  Series RLC Branch3/LConn1 -- Ideal Switch/LConn1
  Series RLC Branch/RConn1 -- Series RLC Branch3/RConn1 -- -/RConn1
  Ideal Switch/RConn1 -- +/RConn1 -- Series RLC Branch/LConn1

== system MPC_SinCasadi_V1_2016b/sm_computation1/Microrred/Microrred/Microrred/Subsystem ==
  Ia_meas : Inport
  Ic_meas : Inport  Port=2
  R_1 : powerlib/Elements/Series RLC Branch  LConnTagsString=__new0  RConnTagsString=__new0  BranchType=R  Resistance=1e6  Inductance=0  SetiL0=off  InitialCurrent=0  Capacitance=0  Setx0=off  InitialVoltage=0  Measurements=None
  R_2 : powerlib/Elements/Series RLC Branch  LConnTagsString=__new0  RConnTagsString=__new0  BranchType=R  Resistance=1e6  Inductance=0  SetiL0=off  InitialCurrent=0  Capacitance=0  Setx0=off  InitialVoltage=0  Measurements=None
  s1 : powerlib/Electrical Sources/Controlled Current Source  Initialize=off  Source_Type=AC  Amplitude=0  Phase=0  Frequency=50  Measurements=None
  s2 : powerlib/Electrical Sources/Controlled Current Source  Initialize=off  Source_Type=AC  Amplitude=0  Phase=0  Frequency=50  Measurements=None
  I_1 : PMIOPort  Side=Right
  I_2 : PMIOPort  Port=2  Side=Right
  wires:
  Ia_meas/1 -> s1/1
  Ic_meas/1 -> s2/1
  connections:
  R_1/RConn1 -- s1/RConn1 -- R_2/RConn1 -- s2/RConn1
  I_1/RConn1 -- R_1/LConn1 -- s1/LConn1
  I_2/RConn1 -- R_2/LConn1 -- s2/LConn1

== matlab function MPC_SinCasadi_V1_2016b/sm_computation1/MPC/MATLAB Function ==
  data: G input; normG output
function normG = fcn(G)

normG = sqrt(trace(G*transpose(G)));

== matlab function MPC_SinCasadi_V1_2016b/sm_computation1/MPC/MPC/MATLAB Function2 ==
  data: gbus input; G output
function G = fcn(gbus)

G = [gbus(1,:), gbus(2,:), gbus(3,:), gbus(4,:)]';
